simulink model "model_sim_CHB9_36pulse_23b"  (R2023b)
settings: Solver=FixedStepAuto  StartTime=0.0  StopTime=0.1  FixedStep=1e-6  RelTol=1e-3
InitFcn:
  | sysinit
values from neighbouring files (symbols this model uses):
  C = 0.03    [sysinit.m]
  L = 0.004    [sysinit.m]
  m = 0.71    [sysinit.m]
  R = 1.2    [sysinit.m]
  st = 5e-7    (= 5e-07)    [sysinit.m]
  Td = 15e-7    (= 1.5e-06)    [sysinit.m]
undefined symbols (not defined in the file or in its folder): f_out
libraries: spsSeriesRLCBranchLib x123, spsDiodeLib x60, spsIGBTLib x48, spsCurrentMeasurementLib x23, spsThreePhaseVIMeasurementLib x13, spsOnDelayLib x12, spsZigzagPhaseShiftingTransformerLib x12, spsUniversalBridgeLib x12, simulink x3, spsMultiWindingTransformerLib x3, spsVoltageMeasurementLib x3, spsThreePhaseProgrammableVoltageSourceLib x1
(part 3 of 3)

== system model_sim_CHB9_36pulse_23b/Subsystem2 ==
  Multi-Winding Transformer36 : spsMultiWindingTransformerLib/Multi-Winding Transformer  LeftWindings=1  RightWindings=10  TappedWindings=no taps  NumberOfTaps=2  SetSaturation=off  Hysteresis=off  DataFile='hysteresis.mat'  Measurements=None  UNITS=pu  NominalPower=[7e6 50]  NominalVoltages="[ 10000  1900 (1-0.2267)/0.6527*1900 0.2267/0.6527*1900 (1-0.5321)/0.7779*1900 0.5321/0.7779*1900 1900*sqrt(3) (1-0.5321)/0.7779*1900 0.5321/0.7779*1900 (1-0.2267)/0.6527*1900 0.2267/0.6527*1900]"  WindingResistances="[ 0.005   0.005 0.005 0.005  0.005  0.005  0.005 0.005 0.005 0.005  0.005]"  WindingInductances="[ 0.02  0.02 0.02  0.02 0.02 0.02  0.02 0.02 0.02 0.02 0.02]"  Rm=50  Lm=50  Saturation=[ 0,0 ; 0.0024,1.2 ; 1.0,1.52 ]  SpecifyInitialFlux=off  InitialFlux=0  BreakLoop=off  DiscreteSolver=Trapezoidal iterative  DataType=off  TransfoNumber=1
      settings: LibrarySourceBlock=|
      | sps_lib/Power Grid Elements/Multi-Winding
      | Transformer
  Multi-Winding Transformer37 : spsMultiWindingTransformerLib/Multi-Winding Transformer  LeftWindings=1  RightWindings=10  TappedWindings=no taps  NumberOfTaps=2  SetSaturation=off  Hysteresis=off  DataFile='hysteresis.mat'  Measurements=None  UNITS=pu  NominalPower=[7e6 50]  NominalVoltages="[ 10000  1900 (1-0.2267)/0.6527*1900 0.2267/0.6527*1900 (1-0.5321)/0.7779*1900 0.5321/0.7779*1900 1900*sqrt(3) (1-0.5321)/0.7779*1900 0.5321/0.7779*1900 (1-0.2267)/0.6527*1900 0.2267/0.6527*1900]"  WindingResistances="[ 0.005   0.005 0.005 0.005  0.005  0.005  0.005 0.005 0.005 0.005  0.005]"  WindingInductances="[ 0.02  0.02 0.02  0.02 0.02 0.02  0.02 0.02 0.02 0.02 0.02]"  Rm=50  Lm=50  Saturation=[ 0,0 ; 0.0024,1.2 ; 1.0,1.52 ]  SpecifyInitialFlux=off  InitialFlux=0  BreakLoop=off  DiscreteSolver=Trapezoidal iterative  DataType=off  TransfoNumber=1
      settings: LibrarySourceBlock=|
      | sps_lib/Power Grid Elements/Multi-Winding
      | Transformer
  Multi-Winding Transformer38 : spsMultiWindingTransformerLib/Multi-Winding Transformer  LeftWindings=1  RightWindings=10  TappedWindings=no taps  NumberOfTaps=2  SetSaturation=off  Hysteresis=off  DataFile='hysteresis.mat'  Measurements=None  UNITS=pu  NominalPower=[7e6 50]  NominalVoltages="[ 10000  1900 (1-0.2267)/0.6527*1900 0.2267/0.6527*1900 (1-0.5321)/0.7779*1900 0.5321/0.7779*1900 1900*sqrt(3) (1-0.5321)/0.7779*1900 0.5321/0.7779*1900 (1-0.2267)/0.6527*1900 0.2267/0.6527*1900]"  WindingResistances="[ 0.005   0.005 0.005 0.005  0.005  0.005  0.005 0.005 0.005 0.005  0.005]"  WindingInductances="[ 0.02  0.02 0.02  0.02 0.02 0.02  0.02 0.02 0.02 0.02 0.02]"  Rm=50  Lm=50  Saturation=[ 0,0 ; 0.0024,1.2 ; 1.0,1.52 ]  SpecifyInitialFlux=off  InitialFlux=0  BreakLoop=off  DiscreteSolver=Trapezoidal iterative  DataType=off  TransfoNumber=1
      settings: LibrarySourceBlock=|
      | sps_lib/Power Grid Elements/Multi-Winding
      | Transformer
  A : PMIOPort  Side=Left
  B : PMIOPort  Port=2  Side=Left
  C : PMIOPort  Port=3  Side=Left
  a-20 : PMIOPort  Port=4  Side=Right
  b-20 : PMIOPort  Port=5  Side=Right
  c-20 : PMIOPort  Port=6  Side=Right
  a10 : PMIOPort  Port=7  Side=Right
  b10 : PMIOPort  Port=8  Side=Right
  c10 : PMIOPort  Port=9  Side=Right
  a-10 : PMIOPort  Port=10  Side=Right
  b-10 : PMIOPort  Port=11  Side=Right
  c-10 : PMIOPort  Port=12  Side=Right
  a20 : PMIOPort  Port=13  Side=Right
  b20 : PMIOPort  Port=14  Side=Right
  c20 : PMIOPort  Port=15  Side=Right
  a0 : PMIOPort  Port=16  Side=Right
  b0 : PMIOPort  Port=17  Side=Right
  c0 : PMIOPort  Port=18  Side=Right
  a30 : PMIOPort  Port=19  Side=Right
  b30 : PMIOPort  Port=20  Side=Right
  c30 : PMIOPort  Port=21  Side=Right
  connections:
  Multi-Winding Transformer38/LConn1 -- C/RConn1
  Multi-Winding Transformer37/RConn1 -- b0/RConn1
  Multi-Winding Transformer36/RConn5 -- a-20/RConn1
  Multi-Winding Transformer36/RConn1 -- a0/RConn1
  Multi-Winding Transformer37/LConn1 -- B/RConn1
  Multi-Winding Transformer37/RConn19 -- b20/RConn1
  Multi-Winding Transformer36/RConn9 -- a-10/RConn1
  Multi-Winding Transformer36/LConn1 -- A/RConn1
  Multi-Winding Transformer37/RConn15 -- b10/RConn1
  Multi-Winding Transformer38/RConn9 -- c-10/RConn1
  Multi-Winding Transformer37/RConn5 -- b-20/RConn1
  Multi-Winding Transformer36/RConn19 -- a20/RConn1
  Multi-Winding Transformer37/RConn9 -- b-10/RConn1
  Multi-Winding Transformer38/RConn13 -- Multi-Winding Transformer37/RConn14 -- Multi-Winding Transformer38/RConn16
  Multi-Winding Transformer38/RConn2 -- Multi-Winding Transformer36/RConn2 -- Multi-Winding Transformer37/RConn2
  Multi-Winding Transformer38/RConn4 -- Multi-Winding Transformer37/RConn3 -- Multi-Winding Transformer37/RConn6
  Multi-Winding Transformer36/RConn15 -- a10/RConn1
  Multi-Winding Transformer37/RConn8 -- Multi-Winding Transformer36/RConn7 -- Multi-Winding Transformer36/RConn10
  Multi-Winding Transformer38/RConn7 -- Multi-Winding Transformer36/RConn8 -- Multi-Winding Transformer38/RConn10
  Multi-Winding Transformer38/RConn19 -- c20/RConn1
  Multi-Winding Transformer38/LConn2 -- Multi-Winding Transformer37/LConn2 -- Multi-Winding Transformer36/LConn2
  b30/RConn1 -- Multi-Winding Transformer36/RConn12 -- Multi-Winding Transformer37/RConn11
  Multi-Winding Transformer38/RConn6 -- Multi-Winding Transformer36/RConn4 -- Multi-Winding Transformer38/RConn3
  Multi-Winding Transformer38/RConn20 -- Multi-Winding Transformer37/RConn18 -- Multi-Winding Transformer38/RConn17
  c30/RConn1 -- Multi-Winding Transformer37/RConn12 -- Multi-Winding Transformer38/RConn11
  Multi-Winding Transformer38/RConn15 -- c10/RConn1
  Multi-Winding Transformer38/RConn8 -- Multi-Winding Transformer37/RConn7 -- Multi-Winding Transformer37/RConn10
  Multi-Winding Transformer38/RConn18 -- Multi-Winding Transformer36/RConn17 -- Multi-Winding Transformer36/RConn20
  Multi-Winding Transformer38/RConn5 -- c-20/RConn1
  Multi-Winding Transformer38/RConn14 -- Multi-Winding Transformer36/RConn13 -- Multi-Winding Transformer36/RConn16
  Multi-Winding Transformer37/RConn13 -- Multi-Winding Transformer36/RConn14 -- Multi-Winding Transformer37/RConn16
  a30/RConn1 -- Multi-Winding Transformer36/RConn11 -- Multi-Winding Transformer38/RConn12
  Multi-Winding Transformer38/RConn1 -- c0/RConn1
  Multi-Winding Transformer36/RConn3 -- Multi-Winding Transformer36/RConn6 -- Multi-Winding Transformer37/RConn4
  Multi-Winding Transformer37/RConn20 -- Multi-Winding Transformer36/RConn18 -- Multi-Winding Transformer37/RConn17

== system model_sim_CHB9_36pulse_23b/Subsystem3 ==
  Zigzag Phase-Shifting Transformer : spsZigzagPhaseShiftingTransformerLib/Zigzag Phase-Shifting Transformer  SecondaryConnection=Delta D1(-30 deg.)  SetSaturation=off  SetInitialFlux=off  Measurements=None  UNITS=pu  NominalPower=[ p 50]  PrimaryVoltage=vp  SecondaryVoltage="[ vs  +5]"  Winding1=windingpri  Winding2=windingpri  Winding3=windingsec  RmLm=mag  Rm=500  Saturation=[ 0,0 ; 0.0024,1.2 ; 1.0,1.52 ]  InitialFluxes=[0,0,0]  BreakLoop=off  DiscreteSolver=Trapezoidal iterative  DataType=off
      settings: LibrarySourceBlock=|
      | sps_lib/Power Grid Elements/Zigzag
      | Phase-Shifting Transformer
  Zigzag Phase-Shifting Transformer1 : spsZigzagPhaseShiftingTransformerLib/Zigzag Phase-Shifting Transformer  SecondaryConnection=Delta D1(-30 deg.)  SetSaturation=off  SetInitialFlux=off  Measurements=None  UNITS=pu  NominalPower=[ p 50]  PrimaryVoltage=vp  SecondaryVoltage="[ vs  +15]"  Winding1=windingpri  Winding2=windingpri  Winding3=windingsec  RmLm=mag  Rm=500  Saturation=[ 0,0 ; 0.0024,1.2 ; 1.0,1.52 ]  InitialFluxes=[0,0,0]  BreakLoop=off  DiscreteSolver=Trapezoidal iterative  DataType=off
      settings: LibrarySourceBlock=|
      | sps_lib/Power Grid Elements/Zigzag
      | Phase-Shifting Transformer
  Zigzag Phase-Shifting Transformer2 : spsZigzagPhaseShiftingTransformerLib/Zigzag Phase-Shifting Transformer  SecondaryConnection=Delta D1(-30 deg.)  SetSaturation=off  SetInitialFlux=off  Measurements=None  UNITS=pu  NominalPower=[ p 50]  PrimaryVoltage=vp  SecondaryVoltage="[ vs  +25]"  Winding1=windingpri  Winding2=windingpri  Winding3=windingsec  RmLm=mag  Rm=500  Saturation=[ 0,0 ; 0.0024,1.2 ; 1.0,1.52 ]  InitialFluxes=[0,0,0]  BreakLoop=off  DiscreteSolver=Trapezoidal iterative  DataType=off
      settings: LibrarySourceBlock=|
      | sps_lib/Power Grid Elements/Zigzag
      | Phase-Shifting Transformer
  Zigzag Phase-Shifting Transformer3 : spsZigzagPhaseShiftingTransformerLib/Zigzag Phase-Shifting Transformer  SecondaryConnection=Delta D1(-30 deg.)  SetSaturation=off  SetInitialFlux=off  Measurements=None  UNITS=pu  NominalPower=[ p 50]  PrimaryVoltage=vp  SecondaryVoltage="[ vs  -25]"  Winding1=windingpri  Winding2=windingpri  Winding3=windingsec  RmLm=mag  Rm=500  Saturation=[ 0,0 ; 0.0024,1.2 ; 1.0,1.52 ]  InitialFluxes=[0,0,0]  BreakLoop=off  DiscreteSolver=Trapezoidal iterative  DataType=off
      settings: LibrarySourceBlock=|
      | sps_lib/Power Grid Elements/Zigzag
      | Phase-Shifting Transformer
  Zigzag Phase-Shifting Transformer4 : spsZigzagPhaseShiftingTransformerLib/Zigzag Phase-Shifting Transformer  SecondaryConnection=Delta D1(-30 deg.)  SetSaturation=off  SetInitialFlux=off  Measurements=None  UNITS=pu  NominalPower=[ p 50]  PrimaryVoltage=vp  SecondaryVoltage="[ vs  -5]"  Winding1=windingpri  Winding2=windingpri  Winding3=windingsec  RmLm=mag  Rm=500  Saturation=[ 0,0 ; 0.0024,1.2 ; 1.0,1.52 ]  InitialFluxes=[0,0,0]  BreakLoop=off  DiscreteSolver=Trapezoidal iterative  DataType=off
      settings: LibrarySourceBlock=|
      | sps_lib/Power Grid Elements/Zigzag
      | Phase-Shifting Transformer
  Zigzag Phase-Shifting Transformer5 : spsZigzagPhaseShiftingTransformerLib/Zigzag Phase-Shifting Transformer  SecondaryConnection=Delta D1(-30 deg.)  SetSaturation=off  SetInitialFlux=off  Measurements=None  UNITS=pu  NominalPower=[ p 50]  PrimaryVoltage=vp  SecondaryVoltage="[ vs  -15]"  Winding1=windingpri  Winding2=windingpri  Winding3=windingsec  RmLm=mag  Rm=500  Saturation=[ 0,0 ; 0.0024,1.2 ; 1.0,1.52 ]  InitialFluxes=[0,0,0]  BreakLoop=off  DiscreteSolver=Trapezoidal iterative  DataType=off
      settings: LibrarySourceBlock=|
      | sps_lib/Power Grid Elements/Zigzag
      | Phase-Shifting Transformer
  A : PMIOPort  Side=Left
  a+5 : PMIOPort  Port=2  Side=Right
  B : PMIOPort  Port=3  Side=Left
  C : PMIOPort  Port=4  Side=Left
  b+5 : PMIOPort  Port=5  Side=Right
  c+5 : PMIOPort  Port=6  Side=Right
  a-25 : PMIOPort  Port=7  Side=Right
  b-25 : PMIOPort  Port=8  Side=Right
  c-25 : PMIOPort  Port=9  Side=Right
  a+15 : PMIOPort  Port=10  Side=Right
  b+15 : PMIOPort  Port=11  Side=Right
  c+15 : PMIOPort  Port=12  Side=Right
  a-15 : PMIOPort  Port=13  Side=Right
  b-15 : PMIOPort  Port=14  Side=Right
  c-15 : PMIOPort  Port=15  Side=Right
  a25 : PMIOPort  Port=16  Side=Right
  b25 : PMIOPort  Port=17  Side=Right
  c25 : PMIOPort  Port=18  Side=Right
  a-5 : PMIOPort  Port=19  Side=Right
  b-5 : PMIOPort  Port=20  Side=Right
  c-5 : PMIOPort  Port=21  Side=Right
  connections:
  Zigzag Phase-Shifting Transformer4/LConn4 -- Zigzag Phase-Shifting Transformer4/LConn5 -- Zigzag Phase-Shifting Transformer4/LConn6
  b+5/RConn1 -- Zigzag Phase-Shifting Transformer/RConn2
  a+5/RConn1 -- Zigzag Phase-Shifting Transformer/RConn1
  c+5/RConn1 -- Zigzag Phase-Shifting Transformer/RConn3
  c-25/RConn1 -- Zigzag Phase-Shifting Transformer3/RConn3
  b-25/RConn1 -- Zigzag Phase-Shifting Transformer3/RConn2
  a-25/RConn1 -- Zigzag Phase-Shifting Transformer3/RConn1
  c+15/RConn1 -- Zigzag Phase-Shifting Transformer1/RConn3
  b+15/RConn1 -- Zigzag Phase-Shifting Transformer1/RConn2
  a+15/RConn1 -- Zigzag Phase-Shifting Transformer1/RConn1
  c-15/RConn1 -- Zigzag Phase-Shifting Transformer5/RConn3
  b-15/RConn1 -- Zigzag Phase-Shifting Transformer5/RConn2
  a-15/RConn1 -- Zigzag Phase-Shifting Transformer5/RConn1
  c25/RConn1 -- Zigzag Phase-Shifting Transformer2/RConn3
  b25/RConn1 -- Zigzag Phase-Shifting Transformer2/RConn2
  a25/RConn1 -- Zigzag Phase-Shifting Transformer2/RConn1
  c-5/RConn1 -- Zigzag Phase-Shifting Transformer4/RConn3
  b-5/RConn1 -- Zigzag Phase-Shifting Transformer4/RConn2
  a-5/RConn1 -- Zigzag Phase-Shifting Transformer4/RConn1
  Zigzag Phase-Shifting Transformer/LConn2 -- Zigzag Phase-Shifting Transformer4/LConn2 -- Zigzag Phase-Shifting Transformer2/LConn2 -- Zigzag Phase-Shifting Transformer5/LConn2 -- Zigzag Phase-Shifting Transformer1/LConn2 -- Zigzag Phase-Shifting Transformer3/LConn2 -- B/RConn1
  C/RConn1 -- Zigzag Phase-Shifting Transformer4/LConn3 -- Zigzag Phase-Shifting Transformer2/LConn3 -- Zigzag Phase-Shifting Transformer5/LConn3 -- Zigzag Phase-Shifting Transformer1/LConn3 -- Zigzag Phase-Shifting Transformer3/LConn3 -- Zigzag Phase-Shifting Transformer/LConn3
  A/RConn1 -- Zigzag Phase-Shifting Transformer4/LConn1 -- Zigzag Phase-Shifting Transformer2/LConn1 -- Zigzag Phase-Shifting Transformer5/LConn1 -- Zigzag Phase-Shifting Transformer1/LConn1 -- Zigzag Phase-Shifting Transformer3/LConn1 -- Zigzag Phase-Shifting Transformer/LConn1
  Zigzag Phase-Shifting Transformer2/LConn4 -- Zigzag Phase-Shifting Transformer2/LConn5 -- Zigzag Phase-Shifting Transformer2/LConn6
  Zigzag Phase-Shifting Transformer5/LConn4 -- Zigzag Phase-Shifting Transformer5/LConn5 -- Zigzag Phase-Shifting Transformer5/LConn6
  Zigzag Phase-Shifting Transformer1/LConn4 -- Zigzag Phase-Shifting Transformer1/LConn5 -- Zigzag Phase-Shifting Transformer1/LConn6
  Zigzag Phase-Shifting Transformer3/LConn4 -- Zigzag Phase-Shifting Transformer3/LConn5 -- Zigzag Phase-Shifting Transformer3/LConn6
  Zigzag Phase-Shifting Transformer/LConn4 -- Zigzag Phase-Shifting Transformer/LConn5 -- Zigzag Phase-Shifting Transformer/LConn6

== system model_sim_CHB9_36pulse_23b/Subsystem4 ==
  Current Measurement : spsCurrentMeasurementLib/Current Measurement  PhasorSimulation=off  OutputType=Complex  PSBequivalent=0
  Voltage Measurement : spsVoltageMeasurementLib/Voltage Measurement  PhasorSimulation=off  OutputType=Complex  PSBequivalent=0
  + : PMIOPort  Side=Left
  - : PMIOPort  Port=2  Side=Left
  +OUT : PMIOPort  Port=3  Side=Right
  -OUT : PMIOPort  Port=4  Side=Right
  tag scope: Idc=global, Udc=global
  wires:
  Current Measurement/1 -> [Idc]
  Voltage Measurement/1 -> [Udc]
  connections:
  Current Measurement/RConn1 -- +OUT/RConn1
  -/RConn1 -- -OUT/RConn1 -- Voltage Measurement/LConn2
  +/RConn1 -- Current Measurement/LConn1 -- Voltage Measurement/LConn1

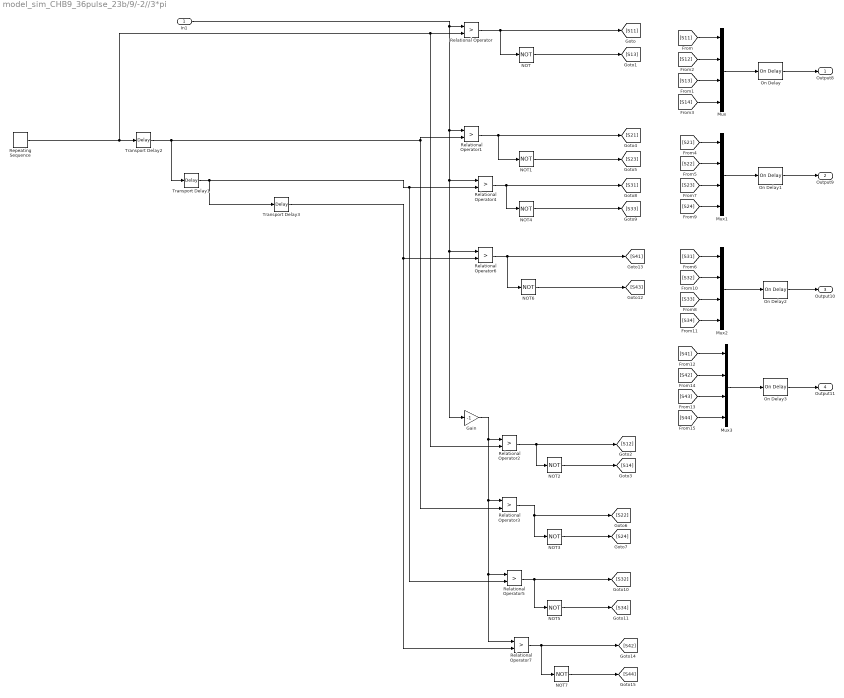
== system model_sim_CHB9_36pulse_23b/9/-2//3*pi ==
  In1 : Inport
  Gain : Gain  Gain=-1
  Mux{,1..3} (4 alike) : Mux
  NOT{,1..7} (8 alike) : Logic  Operator=NOT  AllPortsSameDT=off  OutDataTypeStr=boolean
  On Delay{,1..3} (4 alike) : spsOnDelayLib/On Delay  DelayType=On delay  delay=ttd  ic=0  Ts=0
  Relational Operator{,1..7} (8 alike) : RelationalOperator  Operator=>  OutDataTypeStr=boolean  RndMeth=Simplest  InputSameDT=off
  Repeating Sequence : simulink/Sources/Repeating Sequence  rep_seq_t=[0 0.5 1]/f_car  rep_seq_y=[-1 1 -1]*1000
  Transport Delay1 : TransportDelay  DelayTime=tt/f_car  BufferSize=3072
  Transport Delay2 : TransportDelay  DelayTime=tt/f_car  BufferSize=3072
  Transport Delay3 : TransportDelay  DelayTime=tt/f_car  BufferSize=3072
  Output8 : Outport
  Output9 : Outport  Port=2
  Output10 : Outport  Port=3
  Output11 : Outport  Port=4
  wires:
  On Delay2/1 -> Output10/1
  On Delay1/1 -> Output9/1
  On Delay/1 -> Output8/1
  NOT/1 -> [S13]
  Transport Delay1/1 -> Relational Operator5/2, Relational Operator4/2, Transport Delay3/1
  Transport Delay2/1 -> Transport Delay1/1, Relational Operator3/2, Relational Operator1/2
  [S14] -> Mux/4
  [S23] -> Mux1/3
  [S12] -> Mux/2
  In1/1 -> Relational Operator4/1, Relational Operator6/1, Gain/1, Relational Operator1/1, Relational Operator/1
  [S34] -> Mux2/4
  [S32] -> Mux2/2
  Mux2/1 -> On Delay2/1
  Relational Operator5/1 -> [S32], NOT5/1
  NOT2/1 -> [S14]
  [S21] -> Mux1/1
  NOT4/1 -> [S33]
  Relational Operator1/1 -> NOT1/1, [S21]
  [S22] -> Mux1/2
  [S33] -> Mux2/3
  NOT3/1 -> [S24]
  Mux/1 -> On Delay/1
  Repeating Sequence/1 -> Relational Operator2/2, Relational Operator/2, Transport Delay2/1
  [S24] -> Mux1/4
  Relational Operator4/1 -> [S31], NOT4/1
  Gain/1 -> Relational Operator7/1, Relational Operator5/1, Relational Operator3/1, Relational Operator2/1
  [S13] -> Mux/3
  Relational Operator2/1 -> NOT2/1, [S12]
  [S31] -> Mux2/1
  [S11] -> Mux/1
  NOT5/1 -> [S34]
  Relational Operator/1 -> NOT/1, [S11]
  NOT1/1 -> [S23]
  Mux1/1 -> On Delay1/1
  Relational Operator3/1 -> [S22], NOT3/1
  Relational Operator6/1 -> [S41], NOT6/1
  NOT6/1 -> [S43]
  [S41] -> Mux3/1
  [S43] -> Mux3/3
  Mux3/1 -> On Delay3/1
  On Delay3/1 -> Output11/1
  NOT7/1 -> [S44]
  Relational Operator7/1 -> NOT7/1, [S42]
  Transport Delay3/1 -> Relational Operator7/2, Relational Operator6/2
  [S42] -> Mux3/2
  [S44] -> Mux3/4

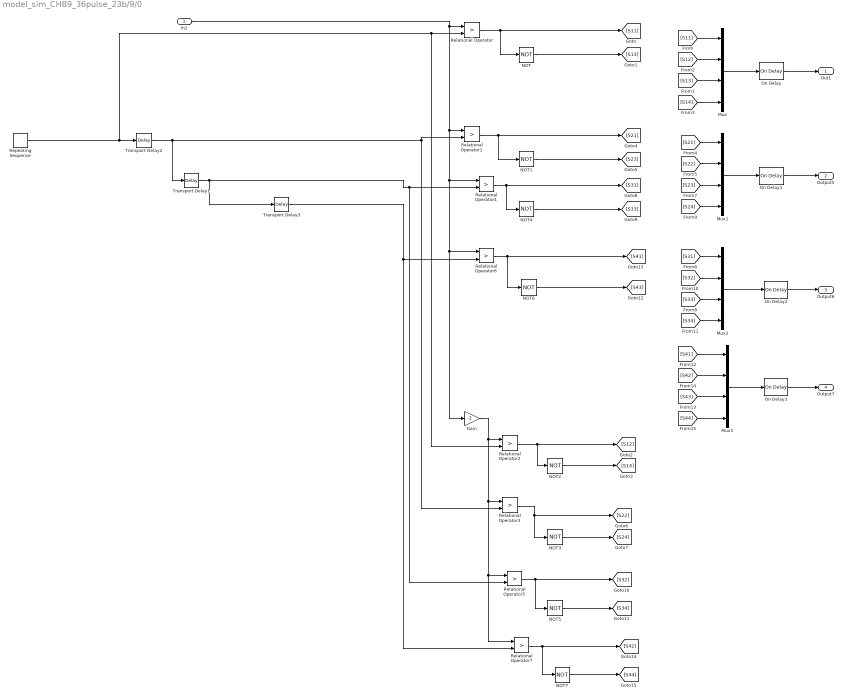
== system model_sim_CHB9_36pulse_23b/9/0 ==
  In1 : Inport
  Gain : Gain  Gain=-1
  Mux{,1..3} (4 alike) : Mux
  NOT{,1..7} (8 alike) : Logic  Operator=NOT  AllPortsSameDT=off  OutDataTypeStr=boolean
  On Delay{,1..3} (4 alike) : spsOnDelayLib/On Delay  DelayType=On delay  delay=ttd  ic=0  Ts=0
  Relational Operator{,1..7} (8 alike) : RelationalOperator  Operator=>  OutDataTypeStr=boolean  RndMeth=Simplest  InputSameDT=off
  Repeating Sequence : simulink/Sources/Repeating Sequence  rep_seq_t=[0 0.5 1]/f_car  rep_seq_y=[-1 1 -1]*1000
  Transport Delay1 : TransportDelay  DelayTime=tt/f_car  BufferSize=3072
  Transport Delay2 : TransportDelay  DelayTime=tt/f_car  BufferSize=3072
  Transport Delay3 : TransportDelay  DelayTime=tt/f_car  BufferSize=3072
  Out1 : Outport
  Output5 : Outport  Port=2
  Output6 : Outport  Port=3
  Output7 : Outport  Port=4
  wires:
  On Delay2/1 -> Output6/1
  On Delay1/1 -> Output5/1
  On Delay/1 -> Out1/1
  NOT/1 -> [S13]
  Transport Delay1/1 -> Relational Operator5/2, Relational Operator4/2, Transport Delay3/1
  Transport Delay2/1 -> Transport Delay1/1, Relational Operator3/2, Relational Operator1/2
  [S14] -> Mux/4
  [S23] -> Mux1/3
  [S12] -> Mux/2
  In1/1 -> Relational Operator4/1, Relational Operator6/1, Gain/1, Relational Operator1/1, Relational Operator/1
  [S34] -> Mux2/4
  [S32] -> Mux2/2
  Mux2/1 -> On Delay2/1
  Relational Operator5/1 -> [S32], NOT5/1
  NOT2/1 -> [S14]
  [S21] -> Mux1/1
  NOT4/1 -> [S33]
  Relational Operator1/1 -> NOT1/1, [S21]
  [S22] -> Mux1/2
  [S33] -> Mux2/3
  NOT3/1 -> [S24]
  Mux/1 -> On Delay/1
  Repeating Sequence/1 -> Relational Operator2/2, Relational Operator/2, Transport Delay2/1
  [S24] -> Mux1/4
  Relational Operator4/1 -> [S31], NOT4/1
  Gain/1 -> Relational Operator7/1, Relational Operator5/1, Relational Operator3/1, Relational Operator2/1
  [S13] -> Mux/3
  Relational Operator2/1 -> NOT2/1, [S12]
  [S31] -> Mux2/1
  [S11] -> Mux/1
  NOT5/1 -> [S34]
  Relational Operator/1 -> NOT/1, [S11]
  NOT1/1 -> [S23]
  Mux1/1 -> On Delay1/1
  Relational Operator3/1 -> [S22], NOT3/1
  Relational Operator6/1 -> [S41], NOT6/1
  NOT6/1 -> [S43]
  [S41] -> Mux3/1
  [S43] -> Mux3/3
  Mux3/1 -> On Delay3/1
  On Delay3/1 -> Output7/1
  NOT7/1 -> [S44]
  Relational Operator7/1 -> NOT7/1, [S42]
  Transport Delay3/1 -> Relational Operator7/2, Relational Operator6/2
  [S42] -> Mux3/2
  [S44] -> Mux3/4

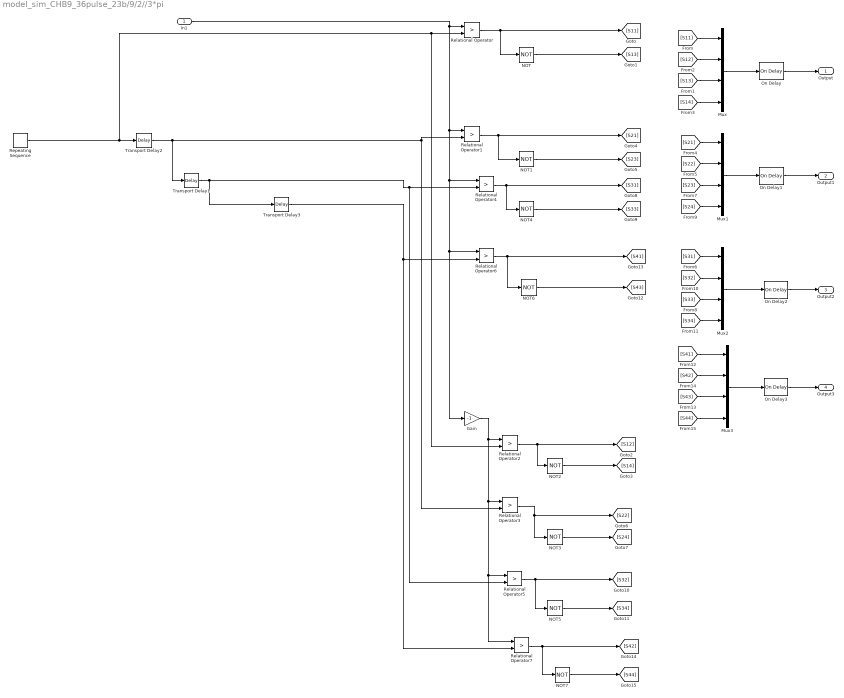
== system model_sim_CHB9_36pulse_23b/9/2//3*pi ==
  In1 : Inport
  Gain : Gain  Gain=-1
  Mux{,1..3} (4 alike) : Mux
  NOT{,1..7} (8 alike) : Logic  Operator=NOT  AllPortsSameDT=off  OutDataTypeStr=boolean
  On Delay{,1..3} (4 alike) : spsOnDelayLib/On Delay  DelayType=On delay  delay=ttd  ic=0  Ts=0
  Relational Operator{,1..7} (8 alike) : RelationalOperator  Operator=>  OutDataTypeStr=boolean  RndMeth=Simplest  InputSameDT=off
  Repeating Sequence : simulink/Sources/Repeating Sequence  rep_seq_t=[0 0.5 1]/f_car  rep_seq_y=[-1 1 -1]*1000
  Transport Delay1 : TransportDelay  DelayTime=tt/f_car  BufferSize=3072
  Transport Delay2 : TransportDelay  DelayTime=tt/f_car  BufferSize=3072
  Transport Delay3 : TransportDelay  DelayTime=tt/f_car  BufferSize=3072
  Output : Outport
  Output1 : Outport  Port=2
  Output2 : Outport  Port=3
  Output3 : Outport  Port=4
  wires:
  On Delay2/1 -> Output2/1
  On Delay1/1 -> Output1/1
  On Delay/1 -> Output/1
  NOT/1 -> [S13]
  Transport Delay1/1 -> Relational Operator5/2, Relational Operator4/2, Transport Delay3/1
  Transport Delay2/1 -> Transport Delay1/1, Relational Operator3/2, Relational Operator1/2
  [S14] -> Mux/4
  [S23] -> Mux1/3
  [S12] -> Mux/2
  In1/1 -> Relational Operator4/1, Relational Operator6/1, Gain/1, Relational Operator1/1, Relational Operator/1
  [S34] -> Mux2/4
  [S32] -> Mux2/2
  Mux2/1 -> On Delay2/1
  Relational Operator5/1 -> [S32], NOT5/1
  NOT2/1 -> [S14]
  [S21] -> Mux1/1
  NOT4/1 -> [S33]
  Relational Operator1/1 -> NOT1/1, [S21]
  [S22] -> Mux1/2
  [S33] -> Mux2/3
  NOT3/1 -> [S24]
  Mux/1 -> On Delay/1
  Repeating Sequence/1 -> Relational Operator2/2, Relational Operator/2, Transport Delay2/1
  [S24] -> Mux1/4
  Relational Operator4/1 -> [S31], NOT4/1
  Gain/1 -> Relational Operator7/1, Relational Operator5/1, Relational Operator3/1, Relational Operator2/1
  [S13] -> Mux/3
  Relational Operator2/1 -> NOT2/1, [S12]
  [S31] -> Mux2/1
  [S11] -> Mux/1
  NOT5/1 -> [S34]
  Relational Operator/1 -> NOT/1, [S11]
  NOT1/1 -> [S23]
  Mux1/1 -> On Delay1/1
  Relational Operator3/1 -> [S22], NOT3/1
  Relational Operator6/1 -> [S41], NOT6/1
  NOT6/1 -> [S43]
  [S41] -> Mux3/1
  [S43] -> Mux3/3
  Mux3/1 -> On Delay3/1
  On Delay3/1 -> Output3/1
  NOT7/1 -> [S44]
  Relational Operator7/1 -> NOT7/1, [S42]
  Transport Delay3/1 -> Relational Operator7/2, Relational Operator6/2
  [S42] -> Mux3/2
  [S44] -> Mux3/4

== system model_sim_CHB9_36pulse_23b/9/Subsystem ==
  In1 : Inport
  In2 : Inport  Port=2
  In3 : Inport  Port=3
  Add{1..3,9} (4 alike) : Sum
  Gain : Gain  Gain=-0.5
  Max : MinMax  Function=max  Inputs=3
  Max1 : MinMax  Inputs=3
  Out1 : Outport
  Out2 : Outport  Port=2
  Out3 : Outport  Port=3
  wires:
  Add3/1 -> Out2/1
  Add2/1 -> Out1/1
  Add9/1 -> Out3/1
  Add1/1 -> Gain/1
  Max1/1 -> Add1/2
  Max/1 -> Add1/1
  Gain/1 -> Add2/1, Add3/1, Add9/1
  In1/1 -> Max/1, Add2/2, Max1/1
  In3/1 -> Max/3, Max1/3, Add9/2
  In2/1 -> Max/2, Max1/2, Add3/2
